simulink model "untitled1"  (R2021b)
settings: Solver=VariableStepAuto  StartTime=0.0  StopTime=2  RelTol=1e-3
settings Model: Creator=Dajun  LastModifiedBy=Dajun

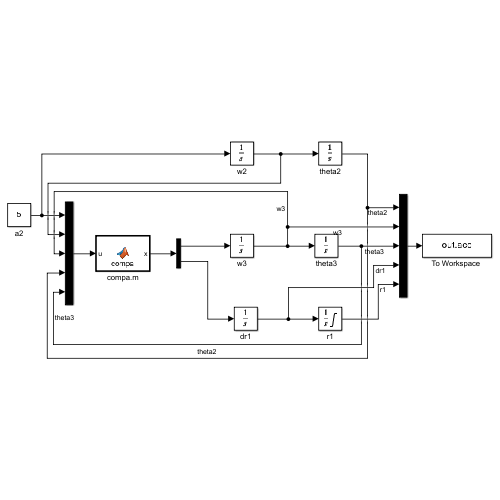
[thumbnail: Simulink's stored preview of the top-level diagram]
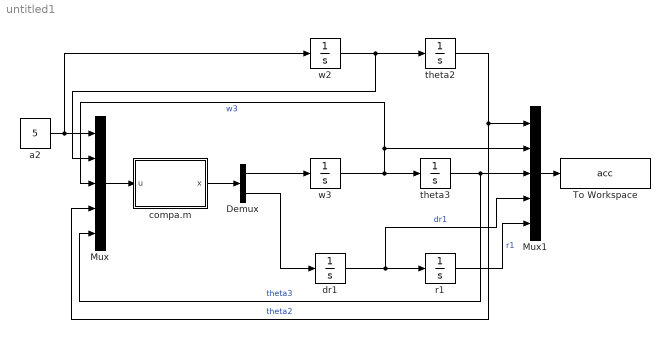
== system untitled1 ==
  Demux : Demux  Outputs=2
  Mux : Mux  Inputs=5
  Mux1 : Mux  Inputs=5
  "To Workspace " : ToWorkspace  VariableName=acc  SampleTime=-1
  a2 : Constant  Value=5
  compa.m : MATLAB Function  TreatAsAtomicUnit=on
  dr1 : Integrator
  r1 : Integrator  InitialCondition=70  LimitOutput=on  UpperSaturationLimit=70  LowerSaturationLimit=40
  theta2 : Integrator
  theta3 : Integrator
  w2 : Integrator
  w3 : Integrator
  wires:
  a2/1 -> w2/1, Mux/1
  Mux/1 -> compa.m/1(u)
  compa.m/1(x) -> Demux/1
  Demux/1 -> w3/1
  Demux/2 -> dr1/1
  w3/1 -> theta3/1, Mux/3, Mux1/2  "w3"
  w2/1 -> Mux/2, theta2/1
  theta2/1 -> Mux/4, Mux1/1  "theta2"
  theta3/1 -> Mux/5, Mux1/3  "theta3"
  dr1/1 -> Mux1/4, r1/1  "dr1"
  r1/1 -> Mux1/5  "r1"
  Mux1/1 -> "To Workspace "/1

== matlab function untitled1/compa.m ==
  data: u input; x output
function x = compa(u)
%u(1) = a2
%u(2) = w2
%u(3) = w3
%u(4) = theta2
%u(5) = theta3
a = zeros(2,2);
b = zeros(2,1);
x = zeros(2,1);
r2 = 15;
r3 = 55;                                     %连杆2、3的长度
a = [r3*sin(u(5)) 1; -r3*cos(u(5)) 0];       %求解运动学方程
% b = [-r2*u(1)*sin(u(2)); r2*u(1)*cos(u(2))];
b = [-r2*cos(u(4))*u(2)^2-r3*cos(u(5))*u(3)^2+r2*sin(u(4))*u(1); r2*cos(u(4))*u(1)-r2*sin(u(4))*u(2)-r3*cos(u(5))*u(3)];
x = inv(a)*b;
